simulink model "Bioloid_HIK_mdl"  (R2013a)
settings: Solver=ode1  StartTime=0  StopTime=inf  FixedStep=0.01  RelTol=1e-3
undefined symbols (not defined in the file or in its folder): Bioloid_HIK
libraries: simulink x30, vrlib x1
settings Model: Creator=root  LastModifiedBy=root

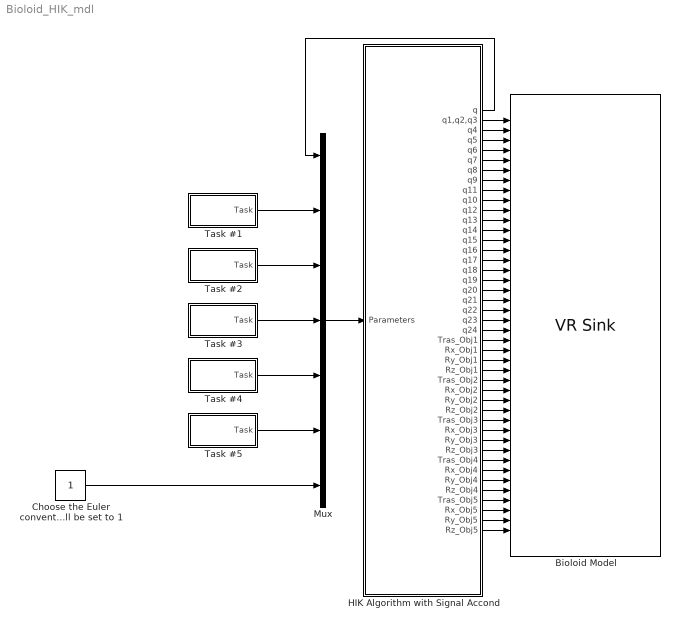
== system Bioloid_HIK_mdl ==
  Bioloid Model : vrlib/VR Sink  InstantiateOnLoad=on  SampleTime=0.1  ViewEnable=on  RemoteChange=off  RemoteView=off  FieldsWritten=TrunkTraslation.translation.3.1.1.double#TrunkRotX.rotation.4.1.1.double#TrunkRotY.rotation.4.1.1.double#TrunkRotZ.rotation.4.1.1.double#Right_Arm.rotation.4.1.1.double#Right_Humeros1.rotation.4.1.1.double#Right_Hand1.rotation.4.1.1.double#Left_Arm.rotation.4.1.1.double#Left_Humeros1.rotation.4.1.1.double#Left_Hand1.rotation.4.1.1.double#Right_Groin.rotation.4.1.1.double#Right_Hip1.rotation.4.1.1.double#Right_Femur1.rotation.4.1.1.double#Right_Tibia1.rotation.4.1.1.double#Right_Ankle1.rotation.4.1.1.double#Right_Foot1.rotation.4.1.1.double#Left_Groin.rotation.4.1.1.double#Left_Hip1.rotation.4.1.1.double#Left_Femur1.rotation.4.1.1.double#Left_Tibia1.rotation.4.1.1.double#Left_Ankle1.rotation.4.1.1.double#Left_Foot1.rotation.4.1.1.double#Obj_1_Tras.translation.3.1.1.double#Obj_1_RotX.rotation.4.1.1.double#Obj_1_RotY.rotation.4.1.1.double#Obj_1_RotZ.rotation.4.1.1.double#Obj_2_Tras.translation.3.1.1.double#Obj_2_RotX.rotation.4.1.1.double#Obj_2_RotY.rotation.4.1.1.double#Obj_2_RotZ.rotation.4.1.1.double#Obj_3_Tras.translation.3.1.1.double#Obj_3_RotX.rotation.4.1.1.double#Obj_3_RotY.rotation.4.1.1.double#Obj_3_RotZ.rotation.4.1.1.double#Obj_4_Tras.translation.3.1.1.double#Obj_4_RotX.rotation.4.1.1.double#Obj_4_RotY.rotation.4.1.1.double#Obj_4_RotZ.rotation.4.1.1.double#Obj_5_Tras.translation.3.1.1.double#Obj_5_RotX.rotation.4.1.1.double#Obj_5_RotY.rotation.4.1.1.double#Obj_5_RotZ.rotation.4.1.1.double  WorldFileName=Bioloid_model_5_obj.wrl  WorldDescription=Bioloid Model for HIK  AutoView=on  VideoDimensions=[]  AllowVariableSize=off
  Choose the Euler convention 1.- XYZ 2.- XZY 3.- XYX 4.- XZX 5.- YXZ 6.- YZX 7.- YXY 8.- YZY 9.- ZXY 10.- ZYX 11.- ZXZ 12.- ZYZ if any other is chosen it will be set to 1 : Constant
  HIK Algorithm with Signal Accond : Subsystem
  Mux : Mux  Inputs=7
  Task #1 : Subsystem
  Task #2 : Subsystem
  Task #3 : Subsystem
  Task #4 : Subsystem
  Task #5 : Subsystem
  wires:
  Task #2/1(Task) -> Mux/3
  Task #1/1(Task) -> Mux/2
  Choose the Euler convention 1.- XYZ 2.- XZY 3.- XYX 4.- XZX 5.- YXZ 6.- YZX 7.- YXY 8.- YZY 9.- ZXY 10.- ZYX 11.- ZXZ 12.- ZYZ if any other is chosen it will be set to 1/1 -> Mux/7
  Mux/1 -> HIK Algorithm with Signal Accond/1(Parameters)
  HIK Algorithm with Signal Accond/1(q) -> Mux/1
  HIK Algorithm with Signal Accond/35(Rz_Obj3) -> Bioloid Model/34
  HIK Algorithm with Signal Accond/6(q7) -> Bioloid Model/5
  HIK Algorithm with Signal Accond/21(q22) -> Bioloid Model/20
  HIK Algorithm with Signal Accond/7(q8) -> Bioloid Model/6
  HIK Algorithm with Signal Accond/37(Rx_Obj4) -> Bioloid Model/36
  HIK Algorithm with Signal Accond/5(q6) -> Bioloid Model/4
  HIK Algorithm with Signal Accond/13(q14) -> Bioloid Model/12
  HIK Algorithm with Signal Accond/25(Rx_Obj1) -> Bioloid Model/24
  HIK Algorithm with Signal Accond/15(q16) -> Bioloid Model/14
  HIK Algorithm with Signal Accond/16(q17) -> Bioloid Model/15
  HIK Algorithm with Signal Accond/12(q13) -> Bioloid Model/11
  HIK Algorithm with Signal Accond/14(q15) -> Bioloid Model/13
  HIK Algorithm with Signal Accond/27(Rz_Obj1) -> Bioloid Model/26
  HIK Algorithm with Signal Accond/42(Ry_Obj5) -> Bioloid Model/41
  HIK Algorithm with Signal Accond/17(q18) -> Bioloid Model/16
  HIK Algorithm with Signal Accond/19(q20) -> Bioloid Model/18
  HIK Algorithm with Signal Accond/18(q19) -> Bioloid Model/17
  HIK Algorithm with Signal Accond/30(Ry_Obj2) -> Bioloid Model/29
  HIK Algorithm with Signal Accond/22(q23) -> Bioloid Model/21
  HIK Algorithm with Signal Accond/39(Rz_Obj4) -> Bioloid Model/38
  HIK Algorithm with Signal Accond/41(Rx_Obj5) -> Bioloid Model/40
  HIK Algorithm with Signal Accond/38(Ry_Obj4) -> Bioloid Model/37
  HIK Algorithm with Signal Accond/33(Rx_Obj3) -> Bioloid Model/32
  HIK Algorithm with Signal Accond/24(Tras_Obj1) -> Bioloid Model/23
  HIK Algorithm with Signal Accond/26(Ry_Obj1) -> Bioloid Model/25
  HIK Algorithm with Signal Accond/8(q9) -> Bioloid Model/7
  HIK Algorithm with Signal Accond/43(Rz_Obj5) -> Bioloid Model/42
  HIK Algorithm with Signal Accond/11(q12) -> Bioloid Model/10
  HIK Algorithm with Signal Accond/32(Tras_Obj3) -> Bioloid Model/31
  HIK Algorithm with Signal Accond/28(Tras_Obj2) -> Bioloid Model/27
  HIK Algorithm with Signal Accond/4(q5) -> Bioloid Model/3
  HIK Algorithm with Signal Accond/34(Ry_Obj3) -> Bioloid Model/33
  HIK Algorithm with Signal Accond/23(q24) -> Bioloid Model/22
  HIK Algorithm with Signal Accond/40(Tras_Obj5) -> Bioloid Model/39
  HIK Algorithm with Signal Accond/10(q10) -> Bioloid Model/9
  HIK Algorithm with Signal Accond/31(Rz_Obj2) -> Bioloid Model/30
  HIK Algorithm with Signal Accond/36(Tras_Obj4) -> Bioloid Model/35
  HIK Algorithm with Signal Accond/9(q11) -> Bioloid Model/8
  HIK Algorithm with Signal Accond/29(Rx_Obj2) -> Bioloid Model/28
  HIK Algorithm with Signal Accond/3(q4) -> Bioloid Model/2
  HIK Algorithm with Signal Accond/2("q1,q2,q3 ") -> Bioloid Model/1
  HIK Algorithm with Signal Accond/20(q21) -> Bioloid Model/19
  Task #3/1(Task) -> Mux/4
  Task #4/1(Task) -> Mux/5
  Task #5/1(Task) -> Mux/6

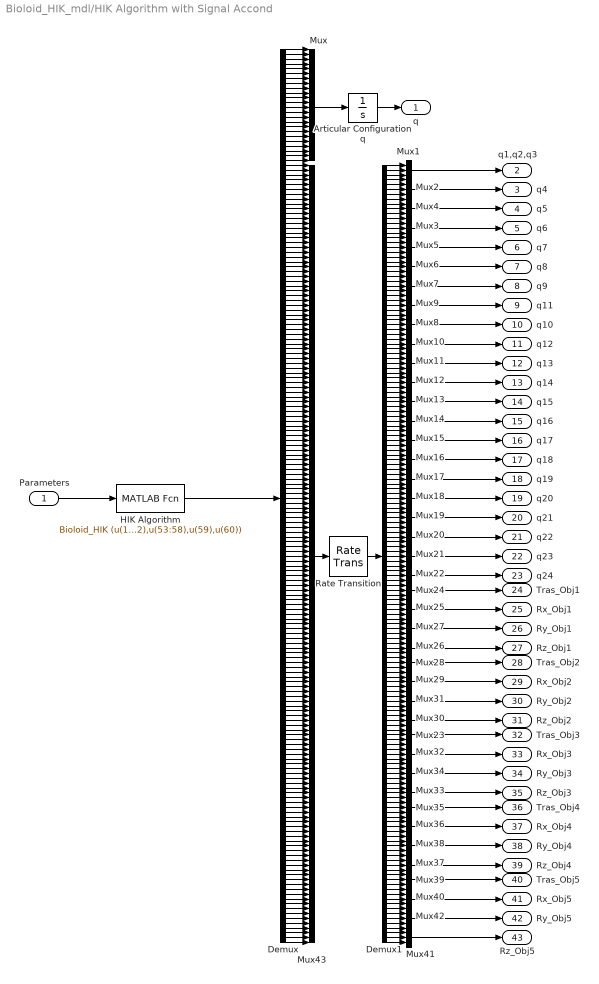
== system Bioloid_HIK_mdl/HIK Algorithm with Signal Accond ==
  Parameters : Inport
  Articular Configuration q : Integrator
  Demux : Demux  Outputs=186
  Demux1 : Demux  Outputs=162
  HIK Algorithm : MATLABFcn  MATLABFcn=Bioloid_HIK (u(1:24),u(25:30),u(31),u(32:37),u(38),u(39:44),u(45),u(46:51),u(52),u(53:58),u(59),u(60))  OutputDimensions=186  SampleTime=0.01
  Mux : Mux  Inputs=24
  Mux{1,23..24,28,35,39} (6 alike) : Mux  Inputs=3
  Mux{2..22,25..27,29..34,36..38,40..42} (36 alike) : Mux
  Mux43 : Mux  Inputs=162
  Rate Transition : RateTransition  OutPortSampleTime=0.1
  q : Outport
  "q1,q2,q3 " : Outport  Port=2
  q4 : Outport  Port=3
  q5 : Outport  Port=4
  q6 : Outport  Port=5
  q7 : Outport  Port=6
  q8 : Outport  Port=7
  q9 : Outport  Port=8
  q11 : Outport  Port=9
  q10 : Outport  Port=10
  q12 : Outport  Port=11
  q13 : Outport  Port=12
  q14 : Outport  Port=13
  q15 : Outport  Port=14
  q16 : Outport  Port=15
  q17 : Outport  Port=16
  q18 : Outport  Port=17
  q19 : Outport  Port=18
  q20 : Outport  Port=19
  q21 : Outport  Port=20
  q22 : Outport  Port=21
  q23 : Outport  Port=22
  q24 : Outport  Port=23
  Tras_Obj1 : Outport  Port=24
  Rx_Obj1 : Outport  Port=25
  Ry_Obj1 : Outport  Port=26
  Rz_Obj1 : Outport  Port=27
  Tras_Obj2 : Outport  Port=28
  Rx_Obj2 : Outport  Port=29
  Ry_Obj2 : Outport  Port=30
  Rz_Obj2 : Outport  Port=31
  Tras_Obj3 : Outport  Port=32
  Rx_Obj3 : Outport  Port=33
  Ry_Obj3 : Outport  Port=34
  Rz_Obj3 : Outport  Port=35
  Tras_Obj4 : Outport  Port=36
  Rx_Obj4 : Outport  Port=37
  Ry_Obj4 : Outport  Port=38
  Rz_Obj4 : Outport  Port=39
  Tras_Obj5 : Outport  Port=40
  Rx_Obj5 : Outport  Port=41
  Ry_Obj5 : Outport  Port=42
  Rz_Obj5 : Outport  Port=43
  wires:
  Parameters/1 -> HIK Algorithm/1
  Articular Configuration q/1 -> q/1
  Demux/2 -> Mux/2
  Demux/8 -> Mux/8
  Demux/1 -> Mux/1
  Demux/3 -> Mux/3
  Demux/7 -> Mux/7
  Demux/11 -> Mux/11
  Demux/9 -> Mux/9
  Demux/6 -> Mux/6
  Demux/10 -> Mux/10
  Demux/23 -> Mux/23
  Demux/20 -> Mux/20
  Demux/21 -> Mux/21
  Demux/14 -> Mux/14
  Demux/22 -> Mux/22
  Demux/13 -> Mux/13
  Demux/19 -> Mux/19
  Demux/18 -> Mux/18
  Demux/16 -> Mux/16
  Demux/15 -> Mux/15
  Demux/17 -> Mux/17
  Demux/12 -> Mux/12
  Demux/5 -> Mux/5
  Demux/4 -> Mux/4
  Demux/24 -> Mux/24
  Mux/1 -> Articular Configuration q/1
  Mux1/1 -> "q1,q2,q3 "/1
  Mux2/1 -> q4/1
  Mux4/1 -> q5/1
  Mux3/1 -> q6/1
  Mux5/1 -> q7/1
  Mux6/1 -> q8/1
  Mux7/1 -> q9/1
  Mux9/1 -> q11/1
  Mux8/1 -> q10/1
  Mux10/1 -> q12/1
  Mux11/1 -> q13/1
  Mux12/1 -> q14/1
  Mux13/1 -> q15/1
  Mux14/1 -> q16/1
  Mux15/1 -> q17/1
  Mux16/1 -> q18/1
  Mux17/1 -> q19/1
  Mux18/1 -> q20/1
  Mux19/1 -> q21/1
  Mux20/1 -> q22/1
  Mux21/1 -> q23/1
  Mux22/1 -> q24/1
  Mux24/1 -> Tras_Obj1/1
  Mux25/1 -> Rx_Obj1/1
  Mux27/1 -> Ry_Obj1/1
  Mux26/1 -> Rz_Obj1/1
  Mux28/1 -> Tras_Obj2/1
  Mux29/1 -> Rx_Obj2/1
  Mux31/1 -> Ry_Obj2/1
  Mux30/1 -> Rz_Obj2/1
  Mux23/1 -> Tras_Obj3/1
  Mux32/1 -> Rx_Obj3/1
  Mux34/1 -> Ry_Obj3/1
  Mux33/1 -> Rz_Obj3/1
  Mux35/1 -> Tras_Obj4/1
  Mux36/1 -> Rx_Obj4/1
  Mux38/1 -> Ry_Obj4/1
  Mux37/1 -> Rz_Obj4/1
  Mux39/1 -> Tras_Obj5/1
  Mux40/1 -> Rx_Obj5/1
  Mux42/1 -> Ry_Obj5/1
  Mux41/1 -> Rz_Obj5/1
  HIK Algorithm/1 -> Demux/1
  Demux/63 -> Mux43/39
  Demux/64 -> Mux43/40
  Demux/65 -> Mux43/41
  Demux/66 -> Mux43/42
  Demux/67 -> Mux43/43
  Demux/68 -> Mux43/44
  Demux/69 -> Mux43/45
  Demux/70 -> Mux43/46
  Demux/72 -> Mux43/48
  Demux/73 -> Mux43/49
  Demux/74 -> Mux43/50
  Demux/75 -> Mux43/51
  Demux/76 -> Mux43/52
  Demux/77 -> Mux43/53
  Demux/78 -> Mux43/54
  Demux/79 -> Mux43/55
  Demux/80 -> Mux43/56
  Demux/81 -> Mux43/57
  Demux/83 -> Mux43/59
  Demux/84 -> Mux43/60
  Demux/85 -> Mux43/61
  Demux/86 -> Mux43/62
  Demux/88 -> Mux43/64
  Demux/89 -> Mux43/65
  Demux/90 -> Mux43/66
  Demux/91 -> Mux43/67
  Demux/92 -> Mux43/68
  Demux/93 -> Mux43/69
  Demux/94 -> Mux43/70
  Demux/95 -> Mux43/71
  Demux/96 -> Mux43/72
  Demux/98 -> Mux43/74
  Demux/99 -> Mux43/75
  Demux/103 -> Mux43/79
  Demux/104 -> Mux43/80
  Demux/105 -> Mux43/81
  Demux/106 -> Mux43/82
  Demux/107 -> Mux43/83
  Demux/108 -> Mux43/84
  Demux/109 -> Mux43/85
  Demux/111 -> Mux43/87
  Demux/112 -> Mux43/88
  Demux/116 -> Mux43/92
  Demux/117 -> Mux43/93
  Demux/118 -> Mux43/94
  Demux/119 -> Mux43/95
  Demux/120 -> Mux43/96
  Demux/121 -> Mux43/97
  Demux/122 -> Mux43/98
  Demux/124 -> Mux43/100
  Demux/125 -> Mux43/101
  Demux/126 -> Mux43/102
  Demux/127 -> Mux43/103
  Demux/128 -> Mux43/104
  Demux/129 -> Mux43/105
  Demux/130 -> Mux43/106
  Demux/131 -> Mux43/107
  Demux/132 -> Mux43/108
  Demux/133 -> Mux43/109
  Demux/135 -> Mux43/111
  Demux/136 -> Mux43/112
  Demux/137 -> Mux43/113
  Demux/138 -> Mux43/114
  Demux/139 -> Mux43/115
  Demux/140 -> Mux43/116
  Demux/141 -> Mux43/117
  Demux/142 -> Mux43/118
  Demux/143 -> Mux43/119
  Demux/25 -> Mux43/1
  Demux/33 -> Mux43/9
  Demux/26 -> Mux43/2
  Demux/36 -> Mux43/12
  Demux/29 -> Mux43/5
  Demux/31 -> Mux43/7
  Demux/30 -> Mux43/6
  Demux/27 -> Mux43/3
  Demux/56 -> Mux43/32
  Demux/34 -> Mux43/10
  Demux/35 -> Mux43/11
  Demux/32 -> Mux43/8
  Demux/61 -> Mux43/37
  Demux/37 -> Mux43/13
  Demux/38 -> Mux43/14
  Demux/40 -> Mux43/16
  Demux/41 -> Mux43/17
  Demux/42 -> Mux43/18
  Demux/43 -> Mux43/19
  Demux/45 -> Mux43/21
  Demux/46 -> Mux43/22
  Demux/47 -> Mux43/23
  Demux/48 -> Mux43/24
  Demux/49 -> Mux43/25
  Demux/51 -> Mux43/27
  Demux/52 -> Mux43/28
  Demux/54 -> Mux43/30
  Demux/55 -> Mux43/31
  Demux/100 -> Mux43/76
  Demux/101 -> Mux43/77
  Demux/102 -> Mux43/78
  Demux/58 -> Mux43/34
  Demux/59 -> Mux43/35
  Demux/113 -> Mux43/89
  Demux/114 -> Mux43/90
  Demux/62 -> Mux43/38
  Demux/57 -> Mux43/33
  Demux/28 -> Mux43/4
  Demux/39 -> Mux43/15
  Demux/50 -> Mux43/26
  Demux/44 -> Mux43/20
  Demux/53 -> Mux43/29
  Demux/123 -> Mux43/99
  Demux/60 -> Mux43/36
  Demux/71 -> Mux43/47
  Demux/134 -> Mux43/110
  Demux/82 -> Mux43/58
  Demux/87 -> Mux43/63
  Demux/97 -> Mux43/73
  Demux/110 -> Mux43/86
  Demux/115 -> Mux43/91
  Demux/144 -> Mux43/120
  Demux/145 -> Mux43/121
  Demux/146 -> Mux43/122
  Demux/147 -> Mux43/123
  Demux/148 -> Mux43/124
  Demux/149 -> Mux43/125
  Demux/150 -> Mux43/126
  Demux/151 -> Mux43/127
  Demux/152 -> Mux43/128
  Demux/153 -> Mux43/129
  Demux/154 -> Mux43/130
  Demux/155 -> Mux43/131
  Demux/156 -> Mux43/132
  Demux/157 -> Mux43/133
  Demux/158 -> Mux43/134
  Demux/159 -> Mux43/135
  Demux/160 -> Mux43/136
  Demux/161 -> Mux43/137
  Demux/162 -> Mux43/138
  Demux/163 -> Mux43/139
  Demux/164 -> Mux43/140
  Demux/165 -> Mux43/141
  Demux/166 -> Mux43/142
  Demux/167 -> Mux43/143
  Demux/168 -> Mux43/144
  Demux/169 -> Mux43/145
  Demux/170 -> Mux43/146
  Demux/171 -> Mux43/147
  Demux/172 -> Mux43/148
  Demux/173 -> Mux43/149
  Demux/174 -> Mux43/150
  Demux/175 -> Mux43/151
  Demux/176 -> Mux43/152
  Demux/177 -> Mux43/153
  Demux/178 -> Mux43/154
  Demux/179 -> Mux43/155
  Demux/180 -> Mux43/156
  Demux/181 -> Mux43/157
  Demux/182 -> Mux43/158
  Demux/183 -> Mux43/159
  Demux/184 -> Mux43/160
  Demux/185 -> Mux43/161
  Demux/186 -> Mux43/162
  Mux43/1 -> Rate Transition/1
  Rate Transition/1 -> Demux1/1
  Demux1/3 -> Mux1/3
  Demux1/101 -> Mux26/3
  Demux1/57 -> Mux15/2
  Demux1/29 -> Mux9/2
  Demux1/30 -> Mux9/3
  Demux1/31 -> Mux9/4
  Demux1/151 -> Mux40/1
  Demux1/152 -> Mux40/2
  Demux1/153 -> Mux40/3
  Demux1/4 -> Mux2/1
  Demux1/154 -> Mux40/4
  Demux1/155 -> Mux42/1
  Demux1/156 -> Mux42/2
  Demux1/8 -> Mux4/1
  Demux1/118 -> Mux23/1
  Demux1/119 -> Mux23/2
  Demux1/120 -> Mux23/3
  Demux1/15 -> Mux3/4
  Demux1/16 -> Mux5/1
  Demux1/109 -> Mux29/4
  Demux1/110 -> Mux31/1
  Demux1/111 -> Mux31/2
  Demux1/7 -> Mux2/4
  Demux1/115 -> Mux30/2
  Demux1/116 -> Mux30/3
  Demux1/117 -> Mux30/4
  Demux1/21 -> Mux6/2
  Demux1/22 -> Mux6/3
  Demux1/130 -> Mux33/2
  Demux1/131 -> Mux33/3
  Demux1/132 -> Mux33/4
  Demux1/59 -> Mux15/4
  Demux1/60 -> Mux16/1
  Demux1/61 -> Mux16/2
  Demux1/17 -> Mux5/2
  Demux1/18 -> Mux5/3
  Demux1/19 -> Mux5/4
  Demux1/20 -> Mux6/1
  Demux1/56 -> Mux15/1
  Demux1/9 -> Mux4/2
  Demux1/23 -> Mux6/4
  Demux1/24 -> Mux7/1
  Demux1/25 -> Mux7/2
  Demux1/86 -> Mux22/3
  Demux1/87 -> Mux22/4
  Demux1/88 -> Mux24/1
  Demux1/124 -> Mux32/4
  Demux1/125 -> Mux34/1
  Demux1/126 -> Mux34/2
  Demux1/11 -> Mux4/4
  Demux1/145 -> Mux37/2
  Demux1/146 -> Mux37/3
  Demux1/147 -> Mux37/4
  Demux1/127 -> Mux34/3
  Demux1/128 -> Mux34/4
  Demux1/129 -> Mux33/1
  Demux1/95 -> Mux27/1
  Demux1/96 -> Mux27/2
  Demux1/97 -> Mux27/3
  Demux1/13 -> Mux3/2
  Demux1/53 -> Mux14/2
  Demux1/54 -> Mux14/3
  Demux1/55 -> Mux14/4
  Demux1/80 -> Mux21/1
  Demux1/81 -> Mux21/2
  Demux1/82 -> Mux21/3
  Demux1/44 -> Mux12/1
  Demux1/45 -> Mux12/2
  Demux1/46 -> Mux12/3
  Demux1/106 -> Mux29/1
  Demux1/107 -> Mux29/2
  Demux1/108 -> Mux29/3
  Demux1/5 -> Mux2/2
  Demux1/47 -> Mux12/4
  Demux1/48 -> Mux13/1
  Demux1/49 -> Mux13/2
  Demux1/89 -> Mux24/2
  Demux1/90 -> Mux24/3
  Demux1/91 -> Mux25/1
  Demux1/157 -> Mux42/3
  Demux1/158 -> Mux42/4
  Demux1/159 -> Mux41/1
  Demux1/58 -> Mux15/3
  Demux1/136 -> Mux36/1
  Demux1/137 -> Mux36/2
  Demux1/138 -> Mux36/3
  Demux1/77 -> Mux20/2
  Demux1/78 -> Mux20/3
  Demux1/79 -> Mux20/4
  Demux1/112 -> Mux31/3
  Demux1/113 -> Mux31/4
  Demux1/114 -> Mux30/1
  Demux1/121 -> Mux32/1
  Demux1/122 -> Mux32/2
  Demux1/123 -> Mux32/3
  Demux1/35 -> Mux8/4
  Demux1/36 -> Mux10/1
  Demux1/37 -> Mux10/2
  Demux1/142 -> Mux38/3
  Demux1/143 -> Mux38/4
  Demux1/144 -> Mux37/1
  Demux1/83 -> Mux21/4
  Demux1/84 -> Mux22/1
  Demux1/85 -> Mux22/2
  Demux1/133 -> Mux35/1
  Demux1/134 -> Mux35/2
  Demux1/135 -> Mux35/3
  Demux1/139 -> Mux36/4
  Demux1/140 -> Mux38/1
  Demux1/141 -> Mux38/2
  Demux1/71 -> Mux18/4
  Demux1/72 -> Mux19/1
  Demux1/73 -> Mux19/2
  Demux1/148 -> Mux39/1
  Demux1/149 -> Mux39/2
  Demux1/150 -> Mux39/3
  Demux1/92 -> Mux25/2
  Demux1/93 -> Mux25/3
  Demux1/94 -> Mux25/4
  Demux1/103 -> Mux28/1
  Demux1/104 -> Mux28/2
  Demux1/105 -> Mux28/3
  Demux1/74 -> Mux19/3
  Demux1/75 -> Mux19/4
  Demux1/76 -> Mux20/1
  Demux1/26 -> Mux7/3
  Demux1/27 -> Mux7/4
  Demux1/28 -> Mux9/1
  Demux1/62 -> Mux16/3
  Demux1/63 -> Mux16/4
  Demux1/64 -> Mux17/1
  Demux1/50 -> Mux13/3
  Demux1/51 -> Mux13/4
  Demux1/52 -> Mux14/1
  Demux1/65 -> Mux17/2
  Demux1/66 -> Mux17/3
  Demux1/67 -> Mux17/4
  Demux1/68 -> Mux18/1
  Demux1/69 -> Mux18/2
  Demux1/70 -> Mux18/3
  Demux1/6 -> Mux2/3
  Demux1/98 -> Mux27/4
  Demux1/99 -> Mux26/1
  Demux1/100 -> Mux26/2
  Demux1/38 -> Mux10/3
  Demux1/39 -> Mux10/4
  Demux1/40 -> Mux11/1
  Demux1/12 -> Mux3/1
  Demux1/41 -> Mux11/2
  Demux1/42 -> Mux11/3
  Demux1/43 -> Mux11/4
  Demux1/2 -> Mux1/2
  Demux1/14 -> Mux3/3
  Demux1/160 -> Mux41/2
  Demux1/161 -> Mux41/3
  Demux1/162 -> Mux41/4
  Demux1/102 -> Mux26/4
  Demux1/10 -> Mux4/3
  Demux1/32 -> Mux8/1
  Demux1/33 -> Mux8/2
  Demux1/34 -> Mux8/3
  Demux1/1 -> Mux1/1

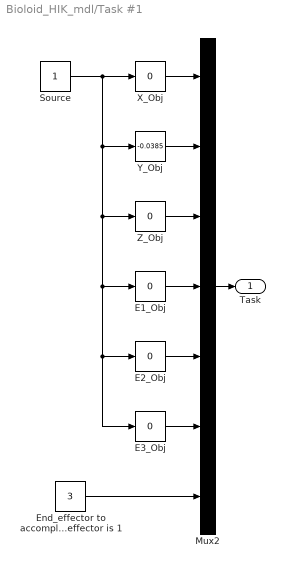
== system Bioloid_HIK_mdl/Task #1 ==
  E1_Obj : simulink/Math Operations/Slider Gain  low=-6.28  gain=0  high=6.28
  E2_Obj : simulink/Math Operations/Slider Gain  low=-6.28  gain=0  high=6.28
  E3_Obj : simulink/Math Operations/Slider Gain  low=-6.28  gain=0  high=6.28
  End_effector to accomplish the task 1.- Right Hand 2- Left Hand 3.- Right Foot 4.- Left Foot 5.- Trunk if another number is choesen the End effector is 1 : Constant  Value=3
  Mux2 : Mux  Inputs=7
  Source : Constant
  X_Obj : simulink/Math Operations/Slider Gain  low=-0.5  gain=0  high=0.5
  Y_Obj : simulink/Math Operations/Slider Gain  low=-0.5  gain=-0.0385  high=0.5
  Z_Obj : simulink/Math Operations/Slider Gain  low=-0.5  gain=0  high=0.5
  Task : Outport
  wires:
  X_Obj/1 -> Mux2/1
  Z_Obj/1 -> Mux2/3
  E1_Obj/1 -> Mux2/4
  E2_Obj/1 -> Mux2/5
  Y_Obj/1 -> Mux2/2
  E3_Obj/1 -> Mux2/6
  End_effector to accomplish the task 1.- Right Hand 2- Left Hand 3.- Right Foot 4.- Left Foot 5.- Trunk if another number is choesen the End effector is 1/1 -> Mux2/7
  Source/1 -> X_Obj/1, Y_Obj/1, Z_Obj/1, E1_Obj/1, E2_Obj/1, E3_Obj/1
  Mux2/1 -> Task/1

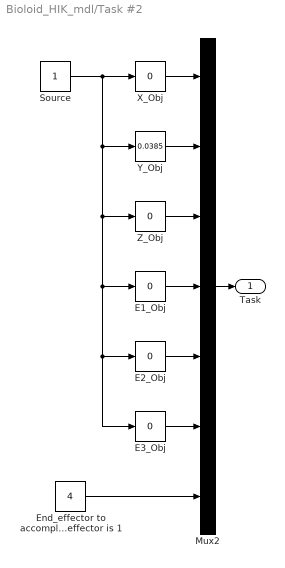
== system Bioloid_HIK_mdl/Task #2 ==
  E1_Obj : simulink/Math Operations/Slider Gain  low=-6.28  gain=0  high=6.28
  E2_Obj : simulink/Math Operations/Slider Gain  low=-6.28  gain=0  high=6.28
  E3_Obj : simulink/Math Operations/Slider Gain  low=-6.28  gain=0  high=6.28
  End_effector to accomplish the task 1.- Right Hand 2- Left Hand 3.- Right Foot 4.- Left Foot 5.- Trunk if another number is choesen the End effector is 1 : Constant  Value=4
  Mux2 : Mux  Inputs=7
  Source : Constant
  X_Obj : simulink/Math Operations/Slider Gain  low=-0.5  gain=0  high=0.5
  Y_Obj : simulink/Math Operations/Slider Gain  low=-0.5  gain=0.0385  high=0.5
  Z_Obj : simulink/Math Operations/Slider Gain  low=-0.5  gain=0  high=0.5
  Task : Outport
  wires:
  X_Obj/1 -> Mux2/1
  Z_Obj/1 -> Mux2/3
  E1_Obj/1 -> Mux2/4
  E2_Obj/1 -> Mux2/5
  Y_Obj/1 -> Mux2/2
  E3_Obj/1 -> Mux2/6
  End_effector to accomplish the task 1.- Right Hand 2- Left Hand 3.- Right Foot 4.- Left Foot 5.- Trunk if another number is choesen the End effector is 1/1 -> Mux2/7
  Source/1 -> X_Obj/1, Y_Obj/1, Z_Obj/1, E1_Obj/1, E2_Obj/1, E3_Obj/1
  Mux2/1 -> Task/1

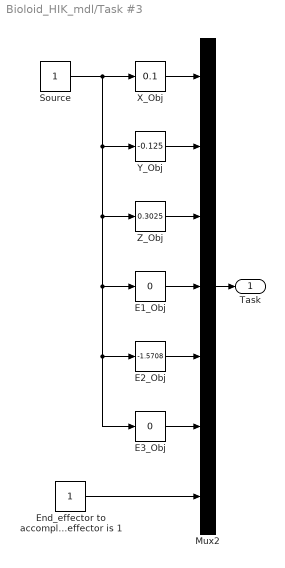
== system Bioloid_HIK_mdl/Task #3 ==
  E1_Obj : simulink/Math Operations/Slider Gain  low=-6.28  gain=0  high=6.28
  E2_Obj : simulink/Math Operations/Slider Gain  low=-6.28  gain=-1.5708  high=6.28
  E3_Obj : simulink/Math Operations/Slider Gain  low=-6.28  gain=0  high=6.28
  End_effector to accomplish the task 1.- Right Hand 2- Left Hand 3.- Right Foot 4.- Left Foot 5.- Trunk if another number is choesen the End effector is 1 : Constant
  Mux2 : Mux  Inputs=7
  Source : Constant
  X_Obj : simulink/Math Operations/Slider Gain  low=-0.5  gain=0.1  high=0.5
  Y_Obj : simulink/Math Operations/Slider Gain  low=-0.5  gain=-0.125  high=0.5
  Z_Obj : simulink/Math Operations/Slider Gain  low=-0.5  gain=0.3025  high=0.5
  Task : Outport
  wires:
  X_Obj/1 -> Mux2/1
  Z_Obj/1 -> Mux2/3
  E1_Obj/1 -> Mux2/4
  E2_Obj/1 -> Mux2/5
  Y_Obj/1 -> Mux2/2
  E3_Obj/1 -> Mux2/6
  End_effector to accomplish the task 1.- Right Hand 2- Left Hand 3.- Right Foot 4.- Left Foot 5.- Trunk if another number is choesen the End effector is 1/1 -> Mux2/7
  Source/1 -> X_Obj/1, Y_Obj/1, Z_Obj/1, E1_Obj/1, E2_Obj/1, E3_Obj/1
  Mux2/1 -> Task/1

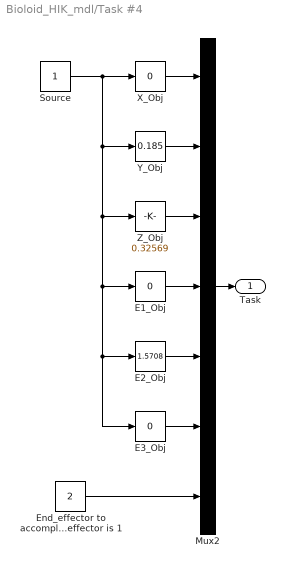
== system Bioloid_HIK_mdl/Task #4 ==
  E1_Obj : simulink/Math Operations/Slider Gain  low=-6.28  gain=0  high=6.28
  E2_Obj : simulink/Math Operations/Slider Gain  low=-6.28  gain=1.5708  high=6.28
  E3_Obj : simulink/Math Operations/Slider Gain  low=-6.28  gain=0  high=6.28
  End_effector to accomplish the task 1.- Right Hand 2- Left Hand 3.- Right Foot 4.- Left Foot 5.- Trunk if another number is choesen the End effector is 1 : Constant  Value=2
  Mux2 : Mux  Inputs=7
  Source : Constant
  X_Obj : simulink/Math Operations/Slider Gain  low=-0.5  gain=0  high=0.5
  Y_Obj : simulink/Math Operations/Slider Gain  low=-0.5  gain=0.185  high=0.5
  Z_Obj : simulink/Math Operations/Slider Gain  low=-0.5  gain=0.32569  high=0.5
  Task : Outport
  wires:
  X_Obj/1 -> Mux2/1
  Z_Obj/1 -> Mux2/3
  E1_Obj/1 -> Mux2/4
  E2_Obj/1 -> Mux2/5
  Y_Obj/1 -> Mux2/2
  E3_Obj/1 -> Mux2/6
  End_effector to accomplish the task 1.- Right Hand 2- Left Hand 3.- Right Foot 4.- Left Foot 5.- Trunk if another number is choesen the End effector is 1/1 -> Mux2/7
  Source/1 -> X_Obj/1, Y_Obj/1, Z_Obj/1, E1_Obj/1, E2_Obj/1, E3_Obj/1
  Mux2/1 -> Task/1

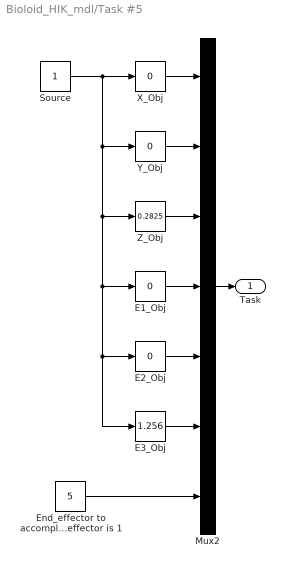
== system Bioloid_HIK_mdl/Task #5 ==
  E1_Obj : simulink/Math Operations/Slider Gain  low=-6.28  gain=0  high=6.28
  E2_Obj : simulink/Math Operations/Slider Gain  low=-6.28  gain=0  high=6.28
  E3_Obj : simulink/Math Operations/Slider Gain  low=-6.28  gain=1.256  high=6.28
  End_effector to accomplish the task 1.- Right Hand 2- Left Hand 3.- Right Foot 4.- Left Foot 5.- Trunk if another number is choesen the End effector is 1 : Constant  Value=5
  Mux2 : Mux  Inputs=7
  Source : Constant
  X_Obj : simulink/Math Operations/Slider Gain  low=-0.5  gain=0  high=0.5
  Y_Obj : simulink/Math Operations/Slider Gain  low=-0.5  gain=0  high=0.5
  Z_Obj : simulink/Math Operations/Slider Gain  low=-0.5  gain=0.2825  high=0.5
  Task : Outport
  wires:
  X_Obj/1 -> Mux2/1
  Z_Obj/1 -> Mux2/3
  E1_Obj/1 -> Mux2/4
  E2_Obj/1 -> Mux2/5
  Y_Obj/1 -> Mux2/2
  E3_Obj/1 -> Mux2/6
  End_effector to accomplish the task 1.- Right Hand 2- Left Hand 3.- Right Foot 4.- Left Foot 5.- Trunk if another number is choesen the End effector is 1/1 -> Mux2/7
  Source/1 -> X_Obj/1, Y_Obj/1, Z_Obj/1, E1_Obj/1, E2_Obj/1, E3_Obj/1
  Mux2/1 -> Task/1
